simulink subsystem "PvtSubSys_AHBC"  (R2020b)
settings: Solver=VariableStepAuto  StartTime=0.0  StopTime=10.0  RelTol=1e-3
undefined symbols (not defined in the file): P_AHBC_ABS_ENABLE, P_AHBC_DRIVE_DIRECTION_ENABLE, P_AHBC_ESP_ENABLE, P_AHBC_FOG_ENABLE, P_AHBC_FOG_TIME, P_AHBC_HIGHBEAM_ACTIVE_GRACE, P_AHBC_LAT_ACC_ENTER, P_AHBC_LAT_ACC_EXIT, P_AHBC_MAX_ONCOMING_DISTANCE_COUPLE2, P_AHBC_MAX_ONCOMING_DISTANCE_ONE2, P_AHBC_MAX_TAILLIGHT_DISTANCE_COUPLE2, P_AHBC_MAX_TAILLIGHT_DISTANCE_ONE2, P_AHBC_SPEED_SWITCH_HIGH_BEAM_OFF2, P_AHBC_SPEED_SWITCH_HIGH_BEAM_ON2, P_AHBC_TrafficStyle, P_AHBC_TURN_LAMP_ENABLE, P_AHBC_WIPER_ENABLE, P_AHBC_WIPER_TIME, P_AHBC_YAW_RATE_ENTER, P_AHBC_YAW_RATE_EXIT
libraries: simulink x57
(part 1 of 4)
settings Model: Creator=GW00184765  LastModifiedBy=GW00204750

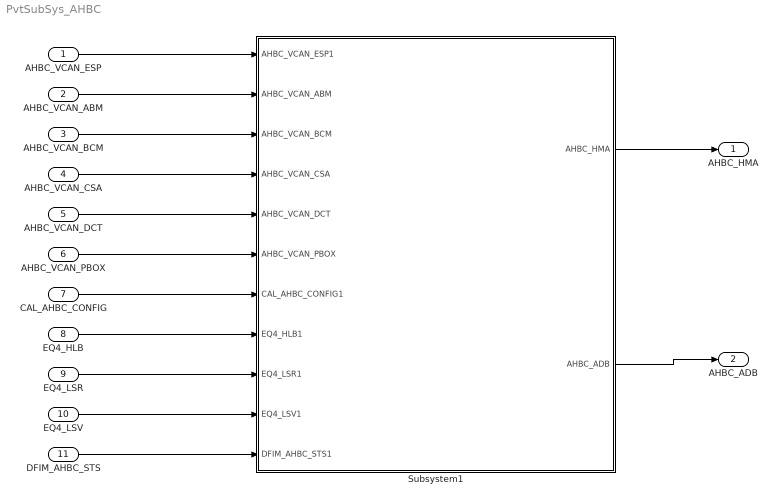
== system PvtSubSys_AHBC ==
  AHBC_VCAN_ESP : Inport  OutDataTypeStr=Bus: VCAN_ESP_MSG_BUS  PortDimensions=1  BusOutputAsStruct=on
  AHBC_VCAN_ABM : Inport  Port=2  OutDataTypeStr=Bus: VCAN_ABM_MSG_BUS  PortDimensions=1  BusOutputAsStruct=on
  AHBC_VCAN_BCM : Inport  Port=3  OutDataTypeStr=Bus: VCAN_BCM_MSG_BUS  PortDimensions=1  BusOutputAsStruct=on
  AHBC_VCAN_CSA : Inport  Port=4  OutDataTypeStr=Bus: VCAN_CSA_MSG_BUS  PortDimensions=1  BusOutputAsStruct=on
  AHBC_VCAN_DCT : Inport  Port=5  OutDataTypeStr=Bus: VCAN_DCT_MSG_BUS  PortDimensions=1  BusOutputAsStruct=on
  AHBC_VCAN_PBOX : Inport  Port=6  OutDataTypeStr=Bus: VCAN_PBOX_MSG_BUS  PortDimensions=1  BusOutputAsStruct=on
  CAL_AHBC_CONFIG : Inport  Port=7  OutDataTypeStr=Bus: CAL_AHBC_CONFIG_BUS  PortDimensions=1  BusOutputAsStruct=on
  EQ4_HLB : Inport  Port=8  OutDataTypeStr=Bus: EQ4_HLB_BUS  PortDimensions=1  BusOutputAsStruct=on
  EQ4_LSR : Inport  Port=9  OutDataTypeStr=Bus: EQ4_LSR_BUS  PortDimensions=1  BusOutputAsStruct=on
  EQ4_LSV : Inport  Port=10  OutDataTypeStr=Bus: EQ4_LSV_BUS  PortDimensions=1  BusOutputAsStruct=on
  DFIM_AHBC_STS : Inport  Port=11  OutDataTypeStr=Bus: DFIM_AHBC_STS_BUS  PortDimensions=1  BusOutputAsStruct=on
  Subsystem1 : Subsystem
  AHBC_HMA : Outport  OutDataTypeStr=Bus: AHBC_HMA_BUS  PortDimensions=1  BusOutputAsStruct=on
  AHBC_ADB : Outport  Port=2  OutDataTypeStr=Bus: AHBC_ADB_BUS  PortDimensions=1  BusOutputAsStruct=on
  wires:
  Subsystem1/2(AHBC_ADB) -> AHBC_ADB/1
  Subsystem1/1(AHBC_HMA) -> AHBC_HMA/1
  AHBC_VCAN_ABM/1 -> Subsystem1/2(AHBC_VCAN_ABM)
  AHBC_VCAN_ESP/1 -> Subsystem1/1(AHBC_VCAN_ESP1)
  AHBC_VCAN_BCM/1 -> Subsystem1/3(AHBC_VCAN_BCM)
  AHBC_VCAN_CSA/1 -> Subsystem1/4(AHBC_VCAN_CSA)
  AHBC_VCAN_DCT/1 -> Subsystem1/5(AHBC_VCAN_DCT)
  AHBC_VCAN_PBOX/1 -> Subsystem1/6(AHBC_VCAN_PBOX)
  CAL_AHBC_CONFIG/1 -> Subsystem1/7(CAL_AHBC_CONFIG1)
  EQ4_HLB/1 -> Subsystem1/8(EQ4_HLB1)
  EQ4_LSR/1 -> Subsystem1/9(EQ4_LSR1)
  EQ4_LSV/1 -> Subsystem1/10(EQ4_LSV1)
  DFIM_AHBC_STS/1 -> Subsystem1/11(DFIM_AHBC_STS1)

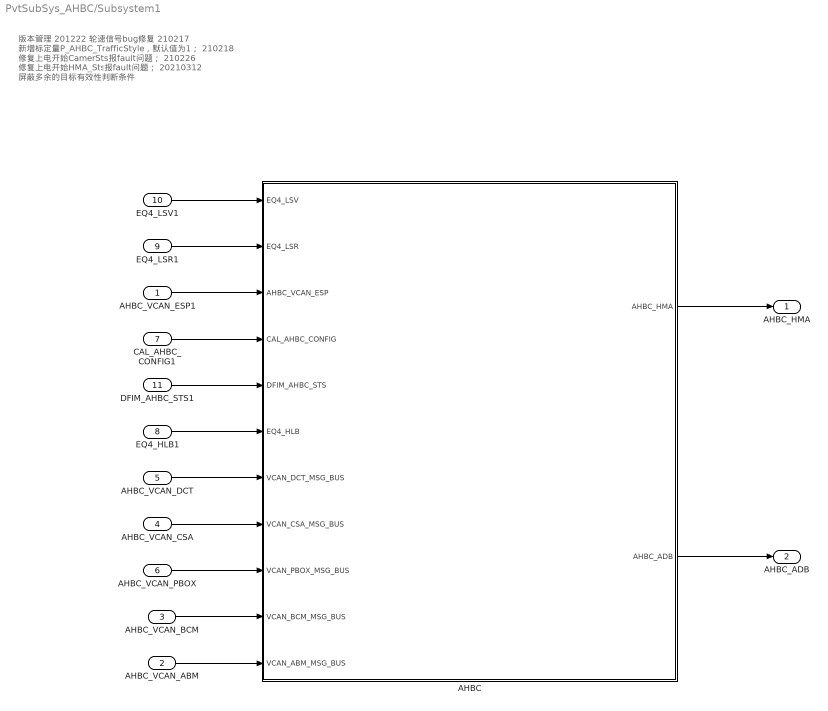
== system PvtSubSys_AHBC/Subsystem1 ==
  note: 版本管理
      | 201222
      | 轮速信号bug修复
      | 210217
      | 新增标定量P_AHBC_TrafficStyle，默认值为1；
      | 210218
      | 修复上电开始CamerSts报fault问题；
      | 210226
      | 修复上电开始HMA_Sts报fault问题；
      | 20210312
      | 屏蔽多余的目标有效性判断条件
  AHBC_VCAN_ESP1 : Inport  OutDataTypeStr=Bus: VCAN_ESP_MSG_BUS  PortDimensions=1  BusOutputAsStruct=on
  AHBC_VCAN_ABM : Inport  Port=2  OutDataTypeStr=Bus: VCAN_ABM_MSG_BUS  PortDimensions=1  BusOutputAsStruct=on
  AHBC_VCAN_BCM : Inport  Port=3  OutDataTypeStr=Bus: VCAN_BCM_MSG_BUS  PortDimensions=1  BusOutputAsStruct=on
  AHBC_VCAN_CSA : Inport  Port=4  OutDataTypeStr=Bus: VCAN_CSA_MSG_BUS  PortDimensions=1  BusOutputAsStruct=on
  AHBC_VCAN_DCT : Inport  Port=5  OutDataTypeStr=Bus: VCAN_DCT_MSG_BUS  PortDimensions=1  BusOutputAsStruct=on
  AHBC_VCAN_PBOX : Inport  Port=6  OutDataTypeStr=Bus: VCAN_PBOX_MSG_BUS  PortDimensions=1  BusOutputAsStruct=on
  CAL_AHBC_CONFIG1 : Inport  Port=7  OutDataTypeStr=Bus: CAL_AHBC_CONFIG_BUS  PortDimensions=1  BusOutputAsStruct=on
  EQ4_HLB1 : Inport  Port=8  OutDataTypeStr=Bus: EQ4_HLB_BUS  PortDimensions=1  BusOutputAsStruct=on
  EQ4_LSR1 : Inport  Port=9  OutDataTypeStr=Bus: EQ4_LSR_BUS  PortDimensions=1  BusOutputAsStruct=on
  EQ4_LSV1 : Inport  Port=10  OutDataTypeStr=Bus: EQ4_LSV_BUS  PortDimensions=1  BusOutputAsStruct=on
  DFIM_AHBC_STS1 : Inport  Port=11  OutDataTypeStr=Bus: DFIM_AHBC_STS_BUS  PortDimensions=1  BusOutputAsStruct=on
  AHBC : Subsystem
  AHBC_HMA : Outport  OutDataTypeStr=Bus: AHBC_HMA_BUS  PortDimensions=1  BusOutputAsStruct=on
  AHBC_ADB : Outport  Port=2  OutDataTypeStr=Bus: AHBC_ADB_BUS  PortDimensions=1  BusOutputAsStruct=on
  wires:
  AHBC/2(AHBC_ADB) -> AHBC_ADB/1
  AHBC/1(AHBC_HMA) -> AHBC_HMA/1
  EQ4_LSV1/1 -> AHBC/1(EQ4_LSV)
  EQ4_LSR1/1 -> AHBC/2(EQ4_LSR)
  EQ4_HLB1/1 -> AHBC/6(EQ4_HLB)
  AHBC_VCAN_ESP1/1 -> AHBC/3(AHBC_VCAN_ESP)
  AHBC_VCAN_ABM/1 -> AHBC/11(VCAN_ABM_MSG_BUS)
  AHBC_VCAN_BCM/1 -> AHBC/10(VCAN_BCM_MSG_BUS)
  AHBC_VCAN_CSA/1 -> AHBC/8(VCAN_CSA_MSG_BUS)
  AHBC_VCAN_DCT/1 -> AHBC/7(VCAN_DCT_MSG_BUS)
  AHBC_VCAN_PBOX/1 -> AHBC/9(VCAN_PBOX_MSG_BUS)
  CAL_AHBC_CONFIG1/1 -> AHBC/4(CAL_AHBC_CONFIG)
  DFIM_AHBC_STS1/1 -> AHBC/5(DFIM_AHBC_STS)

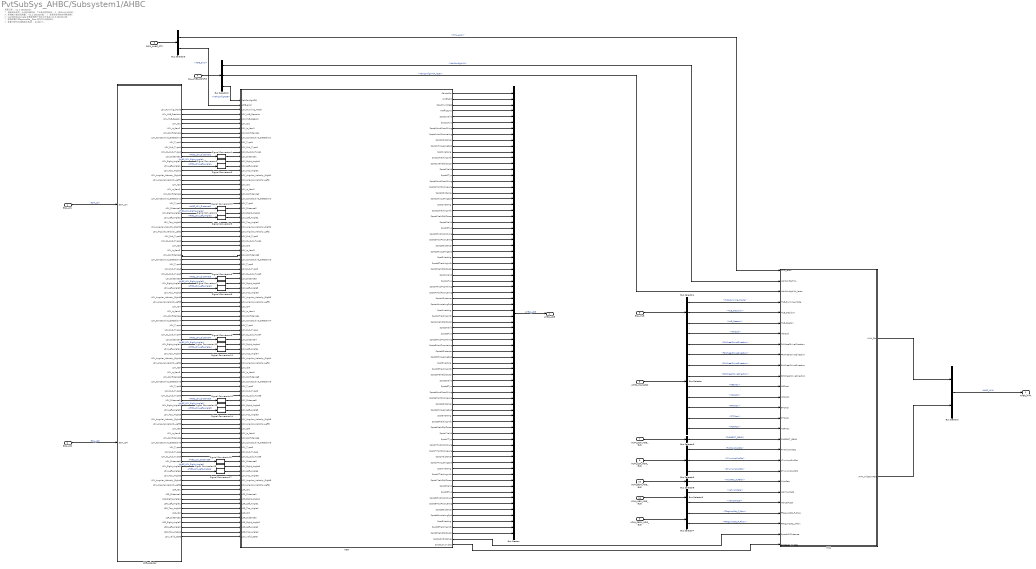
== system PvtSubSys_AHBC/Subsystem1/AHBC ==
  note: 变更记录：
      | V2.1
      | 20201027：
      | 1、调换目标类型，1-6是车辆目标，7-8是反射物目标；
      | 2、修改HMA状态机；
      | 3、新增输入输出观测量；
      | V2.2
      | 20201031：
      | 1、新增目标有效性判断逻辑；
      | 2、LightCtrlParameter字典新增两个自定义的BUS
      | V2.3
      | 20201109：
      | 1、新增后雾灯RFogLmpSts__Pbox信号作为抑制条件；
      | 2、修复行驶方向抑制条件BUG；
      | 210217
      | 新增标定量P_AHBC_TrafficStyle，默认值为1；
      | 210218
      | 修复上电开始CamerSts报fault问题；
      | 210220
      | 优化AmBlight、RoadIllumDetd信号判断逻辑；
      | 210226
      | 修复上电开始HMA_Sts报fault问题；
      | 20210312
      | 屏蔽多余的目标有效性判断条件
  EQ4_LSV : Inport  OutDataTypeStr=Bus: EQ4_LSV_BUS
  EQ4_LSR : Inport  Port=2  OutDataTypeStr=Bus: EQ4_LSR_BUS
  AHBC_VCAN_ESP : Inport  Port=3  OutDataTypeStr=Bus: VCAN_ESP_MSG_BUS  PortDimensions=1  BusOutputAsStruct=on
  CAL_AHBC_CONFIG : Inport  Port=4  OutDataTypeStr=Bus: CAL_AHBC_CONFIG_BUS  PortDimensions=1  BusOutputAsStruct=on
  DFIM_AHBC_STS : Inport  Port=5  OutDataTypeStr=Bus: DFIM_AHBC_STS_BUS  PortDimensions=1  BusOutputAsStruct=on
  EQ4_HLB : Inport  Port=6  OutDataTypeStr=Bus: EQ4_HLB_BUS  PortDimensions=1  BusOutputAsStruct=on
  VCAN_DCT_MSG_BUS : Inport  Port=7  OutDataTypeStr=Bus: VCAN_DCT_MSG_BUS
  VCAN_CSA_MSG_BUS : Inport  Port=8  OutDataTypeStr=Bus: VCAN_CSA_MSG_BUS
  VCAN_PBOX_MSG_BUS : Inport  Port=9  OutDataTypeStr=Bus: VCAN_PBOX_MSG_BUS
  VCAN_BCM_MSG_BUS : Inport  Port=10  OutDataTypeStr=Bus: VCAN_BCM_MSG_BUS
  VCAN_ABM_MSG_BUS : Inport  Port=11  OutDataTypeStr=Bus: VCAN_ABM_MSG_BUS
  ADB : Subsystem
  ADB_adapter : Subsystem
  Bus Creator : BusCreator  Inputs=76  OutDataTypeStr=Bus: AHBC_ADB_BUS
      settings: InheritFromInputs=off
  Bus Creator1 : BusCreator  Inputs=2  OutDataTypeStr=Bus: AHBC_HMA_BUS
  Bus Selector : BusSelector  OutputSignals=VehSpd,FLWheelDriveDirection,FRWheelDriveDirection,RLWheelDriveDirection,RRWheelDriveDirection,ABSActv,VDCActv,BTCActv,PTCActv,MSRActv
  Bus Selector2 : BusSelector  OutputSignals=VehConfigHMA,VehConfigHMA_laser,VehConfigADB
  Bus Selector3 : BusSelector  OutputSignals=HMA_error,ADB_error
  Bus Selector4 : BusSelector  OutputSignals=EQ4_HLB_HDR.HLB_Running_Mode,EQ4_HLB_HDR.HLB_Decision,EQ4_HLB_HDR.HLB_Reason
  Bus Selector5 : BusSelector  OutputSignals=CURRENT_GEAR
  Bus Selector6 : BusSelector  OutputSignals=FrntWiprSwtSts,LTurnLmpSwtSts,RTurnLmpSwtSts
  Bus Selector7 : BusSelector  OutputSignals=FFogLmpSts_F_Pbox,RFogLmpSts_R_Pbox
  Bus Selector8 : BusSelector  OutputSignals=WiprReq_F_PBOX
  Bus Selector9 : BusSelector  OutputSignals=VehYawRate,VehLatAccel
  HMA : Subsystem
  Signal Conversion{1..17,97} (18 alike) : SignalConversion  OverrideOpt=off
  AHBC_HMA : Outport  OutDataTypeStr=Bus: AHBC_HMA_BUS  PortDimensions=1  BusOutputAsStruct=on
  AHBC_ADB : Outport  Port=2  OutDataTypeStr=Bus: AHBC_ADB_BUS  PortDimensions=1  BusOutputAsStruct=on
  wires:
  ADB_adapter/92(LSV_valid_state) -> ADB/94(LSV_valid_state)
  Bus Selector9/2 -> HMA/23(VehLatAccel)  "<VehLatAccel>"
  Bus Selector9/1 -> HMA/22(VehYawRate)  "<VehYawRate>"
  VCAN_ABM_MSG_BUS/1 -> Bus Selector9/1
  Bus Selector8/1 -> HMA/21(WiprReq)  "<WiprReq_F_PBOX>"
  VCAN_BCM_MSG_BUS/1 -> Bus Selector8/1
  Bus Selector7/2 -> HMA/25(RFogLmpSts__Pbox)  "<RFogLmpSts_R_Pbox>"
  Bus Selector7/1 -> HMA/24(FFogLmpSts_F_Pbox)  "<FFogLmpSts_F_Pbox>"
  VCAN_PBOX_MSG_BUS/1 -> Bus Selector7/1
  Bus Selector6/3 -> HMA/20(RTurnLmpSwtSts)  "<RTurnLmpSwtSts>"
  Bus Selector6/2 -> HMA/19(LTurnLmpSwtSts)  "<LTurnLmpSwtSts>"
  Bus Selector6/1 -> HMA/18(FrntWiprSwtSts)  "<FrntWiprSwtSts>"
  VCAN_CSA_MSG_BUS/1 -> Bus Selector6/1
  Bus Selector5/1 -> HMA/17(CURRENT_GEAR)  "<CURRENT_GEAR>"
  VCAN_DCT_MSG_BUS/1 -> Bus Selector5/1
  Signal Conversion17/1 -> ADB/80(LSV_Left_Angle6)
  Signal Conversion16/1 -> ADB/79(LSV_Right_Angle6)
  Signal Conversion15/1 -> ADB/78(LSV_Distance6)
  Signal Conversion14/1 -> ADB/67(LSV_Left_Angle5)
  Signal Conversion13/1 -> ADB/66(LSV_Right_Angle5)
  Signal Conversion12/1 -> ADB/65(LSV_Distance5)
  Signal Conversion11/1 -> ADB/54(LSV_Left_Angle4)
  Signal Conversion10/1 -> ADB/53(LSV_Right_Angle4)
  Signal Conversion9/1 -> ADB/52(LSV_Distance4)
  Signal Conversion8/1 -> ADB/41(LSV_Left_Angle3)
  Signal Conversion7/1 -> ADB/40(LSV_Right_Angle3)
  Signal Conversion6/1 -> ADB/39(LSV_Distance3)
  Signal Conversion5/1 -> ADB/26(LSV_Left_Angle2)
  Signal Conversion4/1 -> ADB/25(LSV_Right_Angle2)
  Signal Conversion3/1 -> ADB/15(LSV_Left_Angle1)
  Signal Conversion2/1 -> ADB/14(LSV_Right_Angle1)
  Signal Conversion1/1 -> ADB/13(LSV_Distance1)
  Signal Conversion97/1 -> ADB/24(LSV_Distance2)
  ADB_adapter/91(LSR_Top_Angle2) -> ADB/93(LSR_Top_Angle2)
  ADB_adapter/90(LSR_Left_Angle2) -> ADB/92(LSR_Left_Angle2)
  ADB_adapter/89(LSR_Right_Angle2) -> ADB/91(LSR_Right_Angle2)
  ADB_adapter/88(LSR_Distance2) -> ADB/90(LSR_Distance2)
  ADB_adapter/87(LSR_ID2) -> ADB/89(LSR_ID2)
  ADB_adapter/86(LSR_Top_Angle1) -> ADB/88(LSR_Top_Angle1)
  ADB_adapter/85(LSR_Left_Angle1) -> ADB/87(LSR_Left_Angle1)
  ADB_adapter/84(LSR_Right_Angle1) -> ADB/86(LSR_Right_Angle1)
  ADB_adapter/83(LSR_Distance1) -> ADB/85(LSR_Distance1)
  ADB_adapter/82(LSR_ID1) -> ADB/84(LSR_ID1)
  ADB_adapter/81(LSV_Angular_Velocity_Left6) -> ADB/83(LSV_Angular_Velocity_Left6)
  ADB_adapter/80(LSV_Angular_Velocity_Right6) -> ADB/82(LSV_Angular_Velocity_Right6)
  ADB_adapter/79(LSV_Top_Angle6) -> ADB/81(LSV_Top_Angle6)
  ADB_adapter/78(LSV_Left_Angle6) -> Signal Conversion17/1  "AHBC_LSV_Left_Angle6"
  ADB_adapter/77(LSV_Right_Angle6) -> Signal Conversion16/1  "AHBC_LSV_Right_Angle6"
  ADB_adapter/76(LSV_Distance6) -> Signal Conversion15/1  "AHBC_LSV_Distance6"
  ADB_adapter/75(LSV_CL_Sub_Type6) -> ADB/77(LSV_CL_Sub_Type6)
  ADB_adapter/74(LSV_Sub_Type6) -> ADB/76(LSV_Sub_Type6)
  ADB_adapter/73(LSV_Type6) -> ADB/75(LSV_Type6)
  ADB_adapter/72(LSV_Consecutive_Detection6) -> ADB/74(LSV_Consecutive_Detection6)
  ADB_adapter/71(LSV_Confidence6) -> ADB/73(LSV_Confidence6)
  ADB_adapter/70(LSV_Is_New6) -> ADB/72(LSV_Is_New6)
  ADB_adapter/69(LSV_ID6) -> ADB/71(LSV_ID6)
  ADB_adapter/68(LSV_Angular_Velocity_Left5) -> ADB/70(LSV_Angular_Velocity_Left5)
  ADB_adapter/67(LSV_Angular_Velocity_Right5) -> ADB/69(LSV_Angular_Velocity_Right5)
  ADB_adapter/66(LSV_Top_Angle5) -> ADB/68(LSV_Top_Angle5)
  ADB_adapter/65(LSV_Left_Angle5) -> Signal Conversion14/1  "AHBC_LSV_Left_Angle5"
  ADB_adapter/64(LSV_Right_Angle5) -> Signal Conversion13/1  "AHBC_LSV_Right_Angle5"
  ADB_adapter/63(LSV_Distance5) -> Signal Conversion12/1  "AHBC_LSV_Distance5"
  ADB_adapter/62(LSV_CL_Sub_Type5) -> ADB/64(LSV_CL_Sub_Type5)
  ADB_adapter/61(LSV_Sub_Type5) -> ADB/63(LSV_Sub_Type5)
  ADB_adapter/60(LSV_Type5) -> ADB/62(LSV_Type5)
  ADB_adapter/59(LSV_Consecutive_Detection5) -> ADB/61(LSV_Consecutive_Detection5)
  ADB_adapter/58(LSV_Confidence5) -> ADB/60(LSV_Confidence5)
  ADB_adapter/57(LSV_Is_New5) -> ADB/59(LSV_Is_New5)
  ADB_adapter/56(LSV_ID5) -> ADB/58(LSV_ID5)
  ADB_adapter/55(LSV_Angular_Velocity_Left4) -> ADB/57(LSV_Angular_Velocity_Left4)
  ADB_adapter/54(LSV_Angular_Velocity_Right4) -> ADB/56(LSV_Angular_Velocity_Right4)
  ADB_adapter/53(LSV_Top_Angle4) -> ADB/55(LSV_Top_Angle4)
  ADB_adapter/52(LSV_Left_Angle4) -> Signal Conversion11/1  "AHBC_LSV_Left_Angle4"
  ADB_adapter/51(LSV_Right_Angle4) -> Signal Conversion10/1  "AHBC_LSV_Right_Angle4"
  ADB_adapter/50(LSV_Distance4) -> Signal Conversion9/1  "AHBC_LSV_Distance4"
  ADB_adapter/49(LSV_CL_Sub_Type4) -> ADB/51(LSV_CL_Sub_Type4)
  ADB_adapter/48(LSV_Sub_Type4) -> ADB/50(LSV_Sub_Type4)
  ADB_adapter/47(LSV_Type4) -> ADB/49(LSV_Type4)
  ADB_adapter/46(LSV_Consecutive_Detection4) -> ADB/48(LSV_Consecutive_Detection4)
  ADB_adapter/45(LSV_Confidence4) -> ADB/47(LSV_Confidence4)
  ADB_adapter/44(LSV_Is_New4) -> ADB/46(LSV_Is_New4)
  ADB_adapter/43(LSV_ID4) -> ADB/45(LSV_ID4)
  ADB_adapter/42(LSV_Angular_Velocity_Left3) -> ADB/44(LSV_Angular_Velocity_Left3)
  ADB_adapter/41(LSV_Angular_Velocity_Right3) -> ADB/43(LSV_Angular_Velocity_Right3)
  ADB_adapter/40(LSV_Top_Angle3) -> ADB/42(LSV_Top_Angle3)
  ADB_adapter/39(LSV_Left_Angle3) -> Signal Conversion8/1  "AHBC_LSV_Left_Angle3"
  ADB_adapter/38(LSV_Right_Angle3) -> Signal Conversion7/1  "AHBC_LSV_Right_Angle3"
  ADB_adapter/37(LSV_Distance3) -> Signal Conversion6/1  "AHBC_LSV_Distance3"
  ADB_adapter/36(LSV_CL_Sub_Type3) -> ADB/38(LSV_CL_Sub_Type3)
  ADB_adapter/35(LSV_Sub_Type3) -> ADB/37(LSV_Sub_Type3)
  ADB_adapter/34(LSV_Type3) -> ADB/36(LSV_Type3)
  ADB_adapter/33(LSV_Consecutive_Detection3) -> ADB/35(LSV_Consecutive_Detection3)
  ADB_adapter/32(LSV_Confidence3) -> ADB/34(LSV_Confidence3)
  ADB_adapter/31(LSV_Is_New3) -> ADB/33(LSV_Is_New3)
  ADB_adapter/30(LSV_ID3) -> ADB/32(LSV_ID3)
  ADB_adapter/29(LSV_CL_Sub_Type2) -> ADB/31(LSV_CL_Sub_Type2)
  ADB_adapter/28(LSV_Sub_Type2) -> ADB/30(LSV_Sub_Type2)
  ADB_adapter/27(LSV_Angular_Velocity_Left2) -> ADB/29(LSV_Angular_Velocity_Left2)
  ADB_adapter/26(LSV_Angular_Velocity_Right2) -> ADB/28(LSV_Angular_Velocity_Right2)
  ADB_adapter/25(LSV_Top_Angle2) -> ADB/27(LSV_Top_Angle2)
  ADB_adapter/24(LSV_Left_Angle2) -> Signal Conversion5/1  "AHBC_LSV_Left_Angle2"
  ADB_adapter/23(LSV_Right_Angle2) -> Signal Conversion4/1  "AHBC_LSV_Right_Angle2"
  ADB_adapter/22(LSV_Distance2) -> Signal Conversion97/1  "AHBC_LSV_Distance2"
  ADB_adapter/21(LSV_Type2) -> ADB/23(LSV_Type2)
  ADB_adapter/20(LSV_Consecutive_Detection2) -> ADB/22(LSV_Consecutive_Detection2)
  ADB_adapter/19(LSV_Confidence2) -> ADB/21(LSV_Confidence2)
  ADB_adapter/18(LSV_Is_New2) -> ADB/20(LSV_Is_New2)
  ADB_adapter/17(LSV_ID2) -> ADB/19(LSV_ID2)
  ADB_adapter/16(LSV_Angular_Velocity_Left1) -> ADB/18(LSV_Angular_Velocity_Left1)
  ADB_adapter/15(LSV_Angular_Velocity_Right1) -> ADB/17(LSV_Angular_Velocity_Right1)
  ADB_adapter/14(LSV_Top_Angle1) -> ADB/16(LSV_Top_Angle1)
  ADB_adapter/13(LSV_Left_Angle1) -> Signal Conversion3/1  "AHBC_LSV_Left_Angle1"
  ADB_adapter/12(LSV_Right_Angle1) -> Signal Conversion2/1  "AHBC_LSV_Right_Angle1"
  ADB_adapter/11(LSV_Distance1) -> Signal Conversion1/1  "AHBC_LSV_Distance1"
  ADB_adapter/10(LSV_CL_Sub_Type1) -> ADB/12(LSV_CL_Sub_Type1)
  ADB_adapter/9(LSV_Sub_Type1) -> ADB/11(LSV_Sub_Type1)
  ADB_adapter/8(LSV_Type1) -> ADB/10(LSV_Type1)
  ADB_adapter/7(LSV_Consecutive_Detection1) -> ADB/9(LSV_Consecutive_Detection1)
  ADB_adapter/6(LSV_Confidence1) -> ADB/8(LSV_Confidence1)
  ADB_adapter/5(LSV_Is_New1) -> ADB/7(LSV_Is_New1)
  ADB_adapter/4(LSV_ID1) -> ADB/6(LSV_ID1)
  ADB_adapter/3(LSV_HLB_Reason) -> ADB/5(LSV_HLB_Reason)
  ADB_adapter/2(LSV_HLB_Decision) -> ADB/4(LSV_HLB_Decision)
  ADB_adapter/1(LSV_Running_Mode) -> ADB/3(LSV_Running_Mode)
  ADB/76(Spots8VehObjClassn) -> Bus Creator/76
  ADB/75(Spots8TrackingInfo) -> Bus Creator/75
  ADB/74(Spot8VertAng) -> Bus Creator/74
  ADB/73(Spots8HozLeAngSpd) -> Bus Creator/73
  ADB/72(Spots8Distance) -> Bus Creator/72
  ADB/71(Spots8HozlPosnLeAng) -> Bus Creator/71
  ADB/70(Spots8HozlPosnRiAng) -> Bus Creator/70
  ADB/69(Spots8Typ) -> Bus Creator/69
  ADB/68(Spots8Valid) -> Bus Creator/68
  ADB/67(Spots7VehObjClassn) -> Bus Creator/67
  ADB/66(Spots7TrackingInfo) -> Bus Creator/66
  ADB/65(Spot7VertAng) -> Bus Creator/65
  ADB/64(Spots7HozLeAngSpd) -> Bus Creator/64
  ADB/63(Spots7Distance) -> Bus Creator/63
  ADB/62(Spots7HozlPosnLeAng) -> Bus Creator/62
  ADB/61(Spots7HozlPosnRiAng) -> Bus Creator/61
  ADB/60(Spots7Typ) -> Bus Creator/60
  ADB/59(Spots7Valid) -> Bus Creator/59
  ADB/58(Spots6VehObjClassn) -> Bus Creator/58
  ADB/57(Spots6TrackingInfo) -> Bus Creator/57
  ADB/56(Spot6VertAng) -> Bus Creator/56
  ADB/55(Spots6HozLeAngSpd) -> Bus Creator/55
  ADB/54(Spots6Distance) -> Bus Creator/54
  ADB/53(Spots6HozlPosnLeAng) -> Bus Creator/53
  ADB/52(Spots6HozlPosnRiAng) -> Bus Creator/52
  ADB/51(Spots6Typ) -> Bus Creator/51
  ADB/50(Spots6Valid) -> Bus Creator/50
  ADB/49(Spots5VehObjClassn) -> Bus Creator/49
  ADB/48(Spots5TrackingInfo) -> Bus Creator/48
  ADB/47(Spot5VertAng) -> Bus Creator/47
  ADB/46(Spots5HozLeAngSpd) -> Bus Creator/46
  ADB/45(Spots5Distance) -> Bus Creator/45
  ADB/44(Spots5HozlPosnLeAng) -> Bus Creator/44
  ADB/43(Spots5HozlPosnRiAng) -> Bus Creator/43
  ADB/42(Spots5Typ) -> Bus Creator/42
  ADB/41(Spots5Valid) -> Bus Creator/41
  ADB/40(Spots4VehObjClassn) -> Bus Creator/40
  ADB/39(Spots4TrackingInfo) -> Bus Creator/39
  ADB/38(Spot4VertAng) -> Bus Creator/38
  ADB/37(Spots4HozLeAngSpd) -> Bus Creator/37
  ADB/36(Spots4Distance) -> Bus Creator/36
  ADB/35(Spots4HozlPosnLeAng) -> Bus Creator/35
  ADB/34(Spots4HozlPosnRiAng) -> Bus Creator/34
  ADB/33(Spots4Typ) -> Bus Creator/33
  ADB/32(Spots4Valid) -> Bus Creator/32
  ADB/31(Spots3VehObjClassn) -> Bus Creator/31
  ADB/30(Spots3TrackingInfo) -> Bus Creator/30
  ADB/29(Spot3VertAng) -> Bus Creator/29
  ADB/28(Spots3HozLeAngSpd) -> Bus Creator/28
  ADB/27(Spots3Distance) -> Bus Creator/27
  ADB/26(Spots3HozlPosnLeAng) -> Bus Creator/26
  ADB/25(Spots3HozlPosnRiAng) -> Bus Creator/25
  ADB/24(Spots3Typ) -> Bus Creator/24
  ADB/23(Spots3Valid) -> Bus Creator/23
  ADB/22(Spots2VehObjClassn) -> Bus Creator/22
  ADB/21(Spots2TrackingInfo) -> Bus Creator/21
  ADB/20(Spot2VertAng) -> Bus Creator/20
  ADB/19(Spots2HozLeAngSpd) -> Bus Creator/19
  ADB/18(Spots2Distance) -> Bus Creator/18
  ADB/17(Spots2HozlPosnLeAng) -> Bus Creator/17
  ADB/16(Spots2HozlPosnRiAng) -> Bus Creator/16
  ADB/15(Spots2Typ) -> Bus Creator/15
  ADB/14(Spots2Valid) -> Bus Creator/14
  ADB/13(Spots1VehObjClassn) -> Bus Creator/13
  ADB/12(Spots1TrackingInfo) -> Bus Creator/12
  ADB/11(Spot1VertAng) -> Bus Creator/11
  ADB/10(Spots1HozLeAngSpd) -> Bus Creator/10
  ADB/9(Spots1Distance) -> Bus Creator/9
  ADB/8(Spots1HozlPosnLeAng) -> Bus Creator/8
  ADB/7(Spots1HozlPosnRiAng) -> Bus Creator/7
  ADB/6(Spots1Typ) -> Bus Creator/6
  ADB/5(Spots1Valid) -> Bus Creator/5
  ADB/4(Trafficstyle) -> Bus Creator/4
  ADB/3(RoadIllumDetd) -> Bus Creator/3
  ADB/2(AmBlight) -> Bus Creator/2
  ADB/1(CamerSts) -> Bus Creator/1
  Bus Selector4/2 -> HMA/5(HLB_Decision)  "<HLB_Decision>"
  Bus Selector4/1 -> HMA/4(HLB_Running_Mode)  "<HLB_Running_Mode>"
  EQ4_HLB/1 -> Bus Selector4/1
  Bus Selector4/3 -> HMA/6(HLB_Reason)  "<HLB_Reason>"
  Bus Selector3/1 -> HMA/1(HMA_error)  "<HMA_error>"
  DFIM_AHBC_STS/1 -> Bus Selector3/1
  Bus Selector2/1 -> HMA/2(VehConfigHMA)  "<VehConfigHMA>"
  Bus Selector2/2 -> HMA/3(VehConfigHMA_laser)  "<VehConfigHMA_laser>"
  CAL_AHBC_CONFIG/1 -> Bus Selector2/1
  Bus Selector/9 -> HMA/15(PTCActv)  "<PTCActv>"
  Bus Selector/8 -> HMA/14(BTCActv)  "<BTCActv>"
  Bus Selector/7 -> HMA/13(VDCActv)  "<VDCActv>"
  Bus Selector/6 -> HMA/12(ABSActv)  "<ABSActv>"
  Bus Selector/10 -> HMA/16(MSRActv)  "<MSRActv>"
  AHBC_VCAN_ESP/1 -> Bus Selector/1
  ADB/78(SpotsLSV_Types) -> HMA/27(SpotsLSV_Types)
  ADB/77(SpotsLSVDistance) -> HMA/26(SpotsLSVDistance)
  Bus Creator1/1 -> AHBC_HMA/1  "AHBC_HMA"
  Bus Creator/1 -> AHBC_ADB/1  "AHBC_ADB"
  Bus Selector/1 -> HMA/7(VehSpd)  "<VehSpd>"
  Bus Selector/5 -> HMA/11(RRWheelDriveDirection)  "<RRWheelDriveDirection>"
  Bus Selector/4 -> HMA/10(RLWheelDriveDirection)  "<RLWheelDriveDirection>"
  Bus Selector/3 -> HMA/9(FRWheelDriveDirection)  "<FRWheelDriveDirection>"
  Bus Selector/2 -> HMA/8(FLWheelDriveDirection)  "<FLWheelDriveDirection>"
  Bus Selector3/2 -> ADB/2(ADB_error)  "<ADB_error>"
  EQ4_LSV/1 -> ADB_adapter/1(EQ4_LSV)  "EQ4_LSV"
  EQ4_LSR/1 -> ADB_adapter/2(EQ4_LSR)  "EQ4_LSR"
  Bus Selector2/3 -> ADB/1(VehConfigADB)  "<VehConfigADB>"
  HMA/2(HMA_HibeamReq) -> Bus Creator1/2
  HMA/1(HMA_Sts) -> Bus Creator1/1

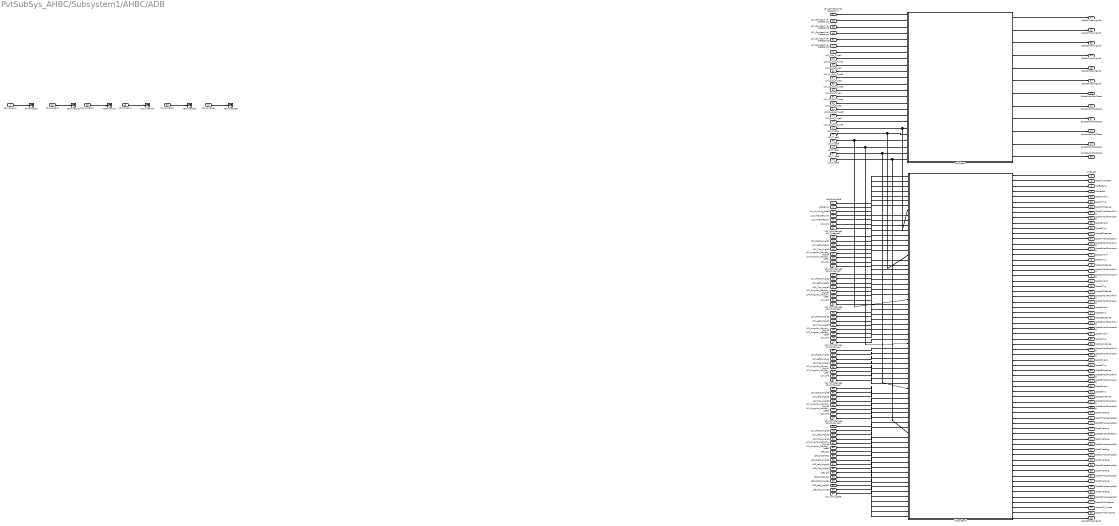
== system PvtSubSys_AHBC/Subsystem1/AHBC/ADB ==
  VehConfigADB : Inport
  ADB_error : Inport  Port=2
  LSV_Running_Mode : Inport  Port=3
  LSV_HLB_Decision : Inport  Port=4
  LSV_HLB_Reason : Inport  Port=5
  LSV_ID1 : Inport  Port=6
  LSV_Is_New1 : Inport  Port=7
  LSV_Confidence1 : Inport  Port=8
  LSV_Consecutive_Detection1 : Inport  Port=9
  LSV_Type1 : Inport  Port=10
  LSV_Sub_Type1 : Inport  Port=11
  LSV_CL_Sub_Type1 : Inport  Port=12
  LSV_Distance1 : Inport  Port=13  OutDataTypeStr=uint16
  LSV_Right_Angle1 : Inport  Port=14
  LSV_Left_Angle1 : Inport  Port=15
  LSV_Top_Angle1 : Inport  Port=16
  LSV_Angular_Velocity_Right1 : Inport  Port=17
  LSV_Angular_Velocity_Left1 : Inport  Port=18
  LSV_ID2 : Inport  Port=19
  LSV_Is_New2 : Inport  Port=20
  LSV_Confidence2 : Inport  Port=21
  LSV_Consecutive_Detection2 : Inport  Port=22
  LSV_Type2 : Inport  Port=23
  LSV_Distance2 : Inport  Port=24  OutDataTypeStr=uint16
  LSV_Right_Angle2 : Inport  Port=25
  LSV_Left_Angle2 : Inport  Port=26
  LSV_Top_Angle2 : Inport  Port=27
  LSV_Angular_Velocity_Right2 : Inport  Port=28
  LSV_Angular_Velocity_Left2 : Inport  Port=29
  LSV_Sub_Type2 : Inport  Port=30
  LSV_CL_Sub_Type2 : Inport  Port=31
  LSV_ID3 : Inport  Port=32
  LSV_Is_New3 : Inport  Port=33
  LSV_Confidence3 : Inport  Port=34
  LSV_Consecutive_Detection3 : Inport  Port=35
  LSV_Type3 : Inport  Port=36
  LSV_Sub_Type3 : Inport  Port=37
  LSV_CL_Sub_Type3 : Inport  Port=38
  LSV_Distance3 : Inport  Port=39  OutDataTypeStr=uint16
  LSV_Right_Angle3 : Inport  Port=40
  LSV_Left_Angle3 : Inport  Port=41
  LSV_Top_Angle3 : Inport  Port=42
  LSV_Angular_Velocity_Right3 : Inport  Port=43
  LSV_Angular_Velocity_Left3 : Inport  Port=44
  LSV_ID4 : Inport  Port=45
  LSV_Is_New4 : Inport  Port=46
  LSV_Confidence4 : Inport  Port=47
  LSV_Consecutive_Detection4 : Inport  Port=48
  LSV_Type4 : Inport  Port=49
  LSV_Sub_Type4 : Inport  Port=50
  LSV_CL_Sub_Type4 : Inport  Port=51
  LSV_Distance4 : Inport  Port=52  OutDataTypeStr=uint16
  LSV_Right_Angle4 : Inport  Port=53
  LSV_Left_Angle4 : Inport  Port=54
  LSV_Top_Angle4 : Inport  Port=55
  LSV_Angular_Velocity_Right4 : Inport  Port=56
  LSV_Angular_Velocity_Left4 : Inport  Port=57
  LSV_ID5 : Inport  Port=58
  LSV_Is_New5 : Inport  Port=59
  LSV_Confidence5 : Inport  Port=60
  LSV_Consecutive_Detection5 : Inport  Port=61
  LSV_Type5 : Inport  Port=62
  LSV_Sub_Type5 : Inport  Port=63
  LSV_CL_Sub_Type5 : Inport  Port=64
  LSV_Distance5 : Inport  Port=65  OutDataTypeStr=uint16
  LSV_Right_Angle5 : Inport  Port=66
  LSV_Left_Angle5 : Inport  Port=67
  LSV_Top_Angle5 : Inport  Port=68
  LSV_Angular_Velocity_Right5 : Inport  Port=69
  LSV_Angular_Velocity_Left5 : Inport  Port=70
  LSV_ID6 : Inport  Port=71
  LSV_Is_New6 : Inport  Port=72
  LSV_Confidence6 : Inport  Port=73
  LSV_Consecutive_Detection6 : Inport  Port=74
  LSV_Type6 : Inport  Port=75
  LSV_Sub_Type6 : Inport  Port=76
  LSV_CL_Sub_Type6 : Inport  Port=77
  LSV_Distance6 : Inport  Port=78  OutDataTypeStr=uint16
  LSV_Right_Angle6 : Inport  Port=79
  LSV_Left_Angle6 : Inport  Port=80
  LSV_Top_Angle6 : Inport  Port=81
  LSV_Angular_Velocity_Right6 : Inport  Port=82
  LSV_Angular_Velocity_Left6 : Inport  Port=83
  LSR_ID1 : Inport  Port=84
  LSR_Distance1 : Inport  Port=85  OutDataTypeStr=uint16
  LSR_Right_Angle1 : Inport  Port=86
  LSR_Left_Angle1 : Inport  Port=87
  LSR_Top_Angle1 : Inport  Port=88
  LSR_ID2 : Inport  Port=89
  LSR_Distance2 : Inport  Port=90  OutDataTypeStr=uint16
  LSR_Right_Angle2 : Inport  Port=91
  LSR_Left_Angle2 : Inport  Port=92
  LSR_Top_Angle2 : Inport  Port=93
  LSV_valid_state : Inport  Port=94
  ObjClassn : Subsystem
  Subsystem1 : Subsystem
  Terminator{3,10,17,24,31,38} (6 alike) : Terminator
  CamerSts : Outport  OutDataTypeStr=uint8  PortDimensions=1
  AmBlight : Outport  Port=2  OutDataTypeStr=boolean  PortDimensions=1
  RoadIllumDetd : Outport  Port=3  OutDataTypeStr=boolean  PortDimensions=1
  Trafficstyle : Outport  Port=4  OutDataTypeStr=uint8  PortDimensions=1
  Spots1Valid : Outport  Port=5  OutDataTypeStr=boolean  PortDimensions=1
  Spots1Typ : Outport  Port=6  OutDataTypeStr=uint8  PortDimensions=1
  Spots1HozlPosnRiAng : Outport  Port=7  OutDataTypeStr=single  PortDimensions=1
  Spots1HozlPosnLeAng : Outport  Port=8  OutDataTypeStr=single  PortDimensions=1
  Spots1Distance : Outport  Port=9  OutDataTypeStr=uint16  PortDimensions=1
  Spots1HozLeAngSpd : Outport  Port=10  OutDataTypeStr=single  PortDimensions=1
  Spot1VertAng : Outport  Port=11  OutDataTypeStr=single  PortDimensions=1
  Spots1TrackingInfo : Outport  Port=12  OutDataTypeStr=boolean  PortDimensions=1
  Spots1VehObjClassn : Outport  Port=13  OutDataTypeStr=uint8  PortDimensions=1
  Spots2Valid : Outport  Port=14  OutDataTypeStr=boolean  PortDimensions=1
  Spots2Typ : Outport  Port=15  OutDataTypeStr=uint8  PortDimensions=1
  Spots2HozlPosnRiAng : Outport  Port=16  OutDataTypeStr=single  PortDimensions=1
  Spots2HozlPosnLeAng : Outport  Port=17  OutDataTypeStr=single  PortDimensions=1
  Spots2Distance : Outport  Port=18  OutDataTypeStr=uint16  PortDimensions=1
  Spots2HozLeAngSpd : Outport  Port=19  OutDataTypeStr=single  PortDimensions=1
  Spot2VertAng : Outport  Port=20  OutDataTypeStr=single  PortDimensions=1
  Spots2TrackingInfo : Outport  Port=21  OutDataTypeStr=boolean  PortDimensions=1
  Spots2VehObjClassn : Outport  Port=22  OutDataTypeStr=uint8  PortDimensions=1
  Spots3Valid : Outport  Port=23  OutDataTypeStr=boolean  PortDimensions=1
  Spots3Typ : Outport  Port=24  OutDataTypeStr=uint8  PortDimensions=1
  Spots3HozlPosnRiAng : Outport  Port=25  OutDataTypeStr=single  PortDimensions=1
  Spots3HozlPosnLeAng : Outport  Port=26  OutDataTypeStr=single  PortDimensions=1
  Spots3Distance : Outport  Port=27  OutDataTypeStr=uint16  PortDimensions=1
  Spots3HozLeAngSpd : Outport  Port=28  OutDataTypeStr=single  PortDimensions=1
  Spot3VertAng : Outport  Port=29  OutDataTypeStr=single  PortDimensions=1
  Spots3TrackingInfo : Outport  Port=30  OutDataTypeStr=boolean  PortDimensions=1
  Spots3VehObjClassn : Outport  Port=31  OutDataTypeStr=uint8  PortDimensions=1
  Spots4Valid : Outport  Port=32  OutDataTypeStr=boolean  PortDimensions=1
  Spots4Typ : Outport  Port=33  OutDataTypeStr=uint8  PortDimensions=1
  Spots4HozlPosnRiAng : Outport  Port=34  OutDataTypeStr=single  PortDimensions=1
  Spots4HozlPosnLeAng : Outport  Port=35  OutDataTypeStr=single  PortDimensions=1
  Spots4Distance : Outport  Port=36  OutDataTypeStr=uint16  PortDimensions=1
  Spots4HozLeAngSpd : Outport  Port=37  OutDataTypeStr=single  PortDimensions=1
  Spot4VertAng : Outport  Port=38  OutDataTypeStr=single  PortDimensions=1
  Spots4TrackingInfo : Outport  Port=39  OutDataTypeStr=boolean  PortDimensions=1
  Spots4VehObjClassn : Outport  Port=40  OutDataTypeStr=uint8  PortDimensions=1
  Spots5Valid : Outport  Port=41  OutDataTypeStr=boolean  PortDimensions=1
  Spots5Typ : Outport  Port=42  OutDataTypeStr=uint8  PortDimensions=1
  Spots5HozlPosnRiAng : Outport  Port=43  OutDataTypeStr=single  PortDimensions=1
  Spots5HozlPosnLeAng : Outport  Port=44  OutDataTypeStr=single  PortDimensions=1
  Spots5Distance : Outport  Port=45  OutDataTypeStr=uint16  PortDimensions=1
  Spots5HozLeAngSpd : Outport  Port=46  OutDataTypeStr=single  PortDimensions=1
  Spot5VertAng : Outport  Port=47  OutDataTypeStr=single  PortDimensions=1
  Spots5TrackingInfo : Outport  Port=48  OutDataTypeStr=boolean  PortDimensions=1
  Spots5VehObjClassn : Outport  Port=49  OutDataTypeStr=uint8  PortDimensions=1
  Spots6Valid : Outport  Port=50  OutDataTypeStr=boolean  PortDimensions=1
  Spots6Typ : Outport  Port=51  OutDataTypeStr=uint8  PortDimensions=1
  Spots6HozlPosnRiAng : Outport  Port=52  OutDataTypeStr=single  PortDimensions=1
  Spots6HozlPosnLeAng : Outport  Port=53  OutDataTypeStr=single  PortDimensions=1
  Spots6Distance : Outport  Port=54  OutDataTypeStr=uint16  PortDimensions=1
  Spots6HozLeAngSpd : Outport  Port=55  OutDataTypeStr=single  PortDimensions=1
  Spot6VertAng : Outport  Port=56  OutDataTypeStr=single  PortDimensions=1
  Spots6TrackingInfo : Outport  Port=57  OutDataTypeStr=boolean  PortDimensions=1
  Spots6VehObjClassn : Outport  Port=58  OutDataTypeStr=uint8  PortDimensions=1
  Spots7Valid : Outport  Port=59  OutDataTypeStr=boolean  PortDimensions=1
  Spots7Typ : Outport  Port=60  OutDataTypeStr=uint8  PortDimensions=1
  Spots7HozlPosnRiAng : Outport  Port=61  OutDataTypeStr=single  PortDimensions=1
  Spots7HozlPosnLeAng : Outport  Port=62  OutDataTypeStr=single  PortDimensions=1
  Spots7Distance : Outport  Port=63  OutDataTypeStr=uint16  PortDimensions=1
  Spots7HozLeAngSpd : Outport  Port=64  OutDataTypeStr=single  PortDimensions=1
  Spot7VertAng : Outport  Port=65  OutDataTypeStr=single  PortDimensions=1
  Spots7TrackingInfo : Outport  Port=66  OutDataTypeStr=boolean  PortDimensions=1
  Spots7VehObjClassn : Outport  Port=67  OutDataTypeStr=uint8  PortDimensions=1
  Spots8Valid : Outport  Port=68  OutDataTypeStr=boolean  PortDimensions=1
  Spots8Typ : Outport  Port=69  OutDataTypeStr=uint8  PortDimensions=1
  Spots8HozlPosnRiAng : Outport  Port=70  OutDataTypeStr=single  PortDimensions=1
  Spots8HozlPosnLeAng : Outport  Port=71  OutDataTypeStr=single  PortDimensions=1
  Spots8Distance : Outport  Port=72  OutDataTypeStr=uint16  PortDimensions=1
  Spots8HozLeAngSpd : Outport  Port=73  OutDataTypeStr=single  PortDimensions=1
  Spot8VertAng : Outport  Port=74  OutDataTypeStr=single  PortDimensions=1
  Spots8TrackingInfo : Outport  Port=75  OutDataTypeStr=boolean  PortDimensions=1
  Spots8VehObjClassn : Outport  Port=76  OutDataTypeStr=uint8  PortDimensions=1
  SpotsLSVDistance : Outport  Port=77  PortDimensions=6
  SpotsLSV_Types : Outport  Port=78  PortDimensions=6
  wires:
  LSV_valid_state/1 -> Subsystem1/70(LSV_valid_state)
  Subsystem1/64(SpotsLSV_Types) -> SpotsLSV_Types/1
  Subsystem1/63(SpotsLSVDistance) -> SpotsLSVDistance/1
  Subsystem1/50(Spots8VehObjClassn) -> Spots8VehObjClassn/1
  Subsystem1/66(Spots8TrackingInfo) -> Spots8TrackingInfo/1
  Subsystem1/49(Spot8VertAng) -> Spot8VertAng/1
  Subsystem1/48(Spots8HozLeAngSpd) -> Spots8HozLeAngSpd/1
  Subsystem1/12(Spots8Distance) -> Spots8Distance/1
  Subsystem1/15(Spots8HozlPosnLeAng) -> Spots8HozlPosnLeAng/1
  Subsystem1/14(Spots8HozlPosnRiAng) -> Spots8HozlPosnRiAng/1
  Subsystem1/11(Spots8Typ) -> Spots8Typ/1
  Subsystem1/10(Spots8Valid) -> Spots8Valid/1
  Subsystem1/13(Spots7VehObjClassn) -> Spots7VehObjClassn/1
  Subsystem1/65(Spots7TrackingInfo) -> Spots7TrackingInfo/1
  Subsystem1/46(Spot7VertAng) -> Spot7VertAng/1
  Subsystem1/47(Spots7HozLeAngSpd) -> Spots7HozLeAngSpd/1
  Subsystem1/7(Spots7Distance) -> Spots7Distance/1
  Subsystem1/9(Spots7HozlPosnLeAng) -> Spots7HozlPosnLeAng/1
  Subsystem1/8(Spots7HozlPosnRiAng) -> Spots7HozlPosnRiAng/1
  Subsystem1/6(Spots7Typ) -> Spots7Typ/1
  Subsystem1/5(Spots7Valid) -> Spots7Valid/1
  ObjClassn/12(Spots6VehObjClassn) -> Spots6VehObjClassn/1
  ObjClassn/6(Spots6TrackingInfo) -> Spots6TrackingInfo/1  "Spots6TrackingInfo"
  Subsystem1/61(Spot6VertAng) -> Spot6VertAng/1
  Subsystem1/62(Spots6HozLeAngSpd) -> Spots6HozLeAngSpd/1
  Subsystem1/43(Spots6Distance) -> Spots6Distance/1
  Subsystem1/45(Spots6HozlPosnLeAng) -> Spots6HozlPosnLeAng/1
  Subsystem1/44(Spots6HozlPosnRiAng) -> Spots6HozlPosnRiAng/1
  Subsystem1/42(Spots6Typ) -> Spots6Typ/1
  Subsystem1/41(Spots6Valid) -> Spots6Valid/1
  ObjClassn/11(Spots5VehObjClassn) -> Spots5VehObjClassn/1
  ObjClassn/5(Spots5TrackingInfo) -> Spots5TrackingInfo/1  "Spots5TrackingInfo"
  Subsystem1/59(Spot5VertAng) -> Spot5VertAng/1
  Subsystem1/60(Spots5HozLeAngSpd) -> Spots5HozLeAngSpd/1
  Subsystem1/40(Spots5HozlPosnLeAng) -> Spots5HozlPosnLeAng/1
  Subsystem1/38(Spots5Distance) -> Spots5Distance/1
  Subsystem1/39(Spots5HozlPosnRiAng) -> Spots5HozlPosnRiAng/1
  Subsystem1/37(Spots5Typ) -> Spots5Typ/1
  Subsystem1/36(Spots5Valid) -> Spots5Valid/1
  Subsystem1/2(RoadIllumDetd) -> RoadIllumDetd/1
  Subsystem1/1(AmBlight) -> AmBlight/1
  ObjClassn/10(Spots4VehObjClassn) -> Spots4VehObjClassn/1
  ObjClassn/4(Spots4TrackingInfo) -> Spots4TrackingInfo/1  "Spots4TrackingInfo"
  Subsystem1/58(Spots4HozLeAngSpd) -> Spots4HozLeAngSpd/1
  Subsystem1/57(Spot4VertAng) -> Spot4VertAng/1
  Subsystem1/33(Spots4Distance) -> Spots4Distance/1
  Subsystem1/35(Spots4HozlPosnLeAng) -> Spots4HozlPosnLeAng/1
  Subsystem1/34(Spots4HozlPosnRiAng) -> Spots4HozlPosnRiAng/1
  Subsystem1/32(Spots4Typ) -> Spots4Typ/1
  Subsystem1/31(Spots4Valid) -> Spots4Valid/1
  ObjClassn/9(Spots3VehObjClassn) -> Spots3VehObjClassn/1
  ObjClassn/3(Spots3TrackingInfo) -> Spots3TrackingInfo/1  "Spots3TrackingInfo"
  Subsystem1/55(Spot3VertAng) -> Spot3VertAng/1
  Subsystem1/56(Spots3HozLeAngSpd) -> Spots3HozLeAngSpd/1
  Subsystem1/28(Spots3Distance) -> Spots3Distance/1
  Subsystem1/30(Spots3HozlPosnLeAng) -> Spots3HozlPosnLeAng/1
  Subsystem1/29(Spots3HozlPosnRiAng) -> Spots3HozlPosnRiAng/1
  Subsystem1/27(Spots3Typ) -> Spots3Typ/1
  Subsystem1/26(Spots3Valid) -> Spots3Valid/1
  ObjClassn/8(Spots2VehObjClassn) -> Spots2VehObjClassn/1
  ObjClassn/2(Spots2TrackingInfo) -> Spots2TrackingInfo/1  "Spots2TrackingInfo"
  Subsystem1/53(Spot2VertAng) -> Spot2VertAng/1
  Subsystem1/54(Spots2HozLeAngSpd) -> Spots2HozLeAngSpd/1
  Subsystem1/23(Spots2Distance) -> Spots2Distance/1
  Subsystem1/25(Spots2HozlPosnLeAng) -> Spots2HozlPosnLeAng/1
  Subsystem1/24(Spots2HozlPosnRiAng) -> Spots2HozlPosnRiAng/1
  Subsystem1/22(Spots2Typ) -> Spots2Typ/1
  Subsystem1/21(Spots2Valid) -> Spots2Valid/1
  Subsystem1/20(Spots1HozlPosnLeAng) -> Spots1HozlPosnLeAng/1
  Subsystem1/19(Spots1HozlPosnRiAng) -> Spots1HozlPosnRiAng/1
  Subsystem1/18(Spots1Distance) -> Spots1Distance/1
  Subsystem1/17(Spots1Typ) -> Spots1Typ/1
  Subsystem1/16(Spots1Valid) -> Spots1Valid/1
  ObjClassn/7(Spots1VehObjClassn) -> Spots1VehObjClassn/1
  ObjClassn/1(Spots1TrackingInfo) -> Spots1TrackingInfo/1  "Spots1TrackingInfo"
  Subsystem1/51(Spot1VertAng) -> Spot1VertAng/1
  Subsystem1/52(Spots1HozLeAngSpd) -> Spots1HozLeAngSpd/1
  Subsystem1/4(CamerSts) -> CamerSts/1
  Subsystem1/3(TrafficStyle) -> Trafficstyle/1
  LSV_Consecutive_Detection5/1 -> ObjClassn/5(LSV_Consecutive_Detection5)
  LSV_Consecutive_Detection2/1 -> ObjClassn/2(LSV_Consecutive_Detection2)
  LSV_Type2/1 -> Subsystem1/17(LSV_Type2), ObjClassn/20(LSV_Type2)
  LSV_Angular_Velocity_Right6/1 -> Subsystem1/58(LSV_Angular_Velocity_Right6)
  LSV_Left_Angle5/1 -> Subsystem1/47(LSV_Left_Angle5)
  LSV_Right_Angle4/1 -> Subsystem1/37(LSV_Right_Angle4)
  LSV_Sub_Type4/1 -> ObjClassn/13(LSV_Sub_Type4)
  LSV_Top_Angle6/1 -> Subsystem1/57(LSV_Top_Angle6)
  LSV_Angular_Velocity_Left1/1 -> Subsystem1/14(LSV_Angular_Velocity_Left1)
  LSV_CL_Sub_Type4/1 -> ObjClassn/14(LSV_CL_Sub_Type4)
  LSV_Distance6/1 -> Subsystem1/54(LSV_Distance6)
  LSV_Angular_Velocity_Right3/1 -> Subsystem1/31(LSV_Angular_Velocity_Right3)
  LSV_Consecutive_Detection6/1 -> ObjClassn/6(LSV_Consecutive_Detection6)
  LSV_Type6/1 -> Subsystem1/53(LSV_Type6), ObjClassn/24(LSV_Type6)
  LSV_Type1/1 -> Subsystem1/8(LSV_Type1), ObjClassn/19(LSV_Type1)
  LSV_Sub_Type5/1 -> ObjClassn/15(LSV_Sub_Type5)
  LSV_Angular_Velocity_Right5/1 -> Subsystem1/49(LSV_Angular_Velocity_Right5)
  LSV_Consecutive_Detection1/1 -> ObjClassn/1(LSV_Consecutive_Detection1)
  LSR_Distance2/1 -> Subsystem1/66(LSR_Distance2)
  LSV_Top_Angle4/1 -> Subsystem1/39(LSV_Top_Angle4)
  LSV_Angular_Velocity_Right4/1 -> Subsystem1/40(LSV_Angular_Velocity_Right4)
  LSR_Right_Angle2/1 -> Subsystem1/67(LSR_Right_Angle2)
  LSV_Is_New2/1 -> Terminator10/1
  LSR_Top_Angle1/1 -> Subsystem1/64(LSR_Top_Angle1)
  LSV_Angular_Velocity_Left6/1 -> Subsystem1/59(LSV_Angular_Velocity_Left6)
  LSR_ID2/1 -> Subsystem1/65(LSR_ID2)
  LSV_ID6/1 -> Subsystem1/51(LSV_ID6)
  LSV_CL_Sub_Type5/1 -> ObjClassn/16(LSV_CL_Sub_Type5)
  LSV_Right_Angle6/1 -> Subsystem1/55(LSV_Right_Angle6)
  LSR_Left_Angle1/1 -> Subsystem1/63(LSR_Left_Angle1)
  LSV_Left_Angle6/1 -> Subsystem1/56(LSV_Left_Angle6)
  ADB_error/1 -> Subsystem1/2(ADB_error)
  LSV_Distance5/1 -> Subsystem1/45(LSV_Distance5)
  LSV_Distance4/1 -> Subsystem1/36(LSV_Distance4)
  LSV_ID4/1 -> Subsystem1/33(LSV_ID4)
  LSV_Type5/1 -> Subsystem1/44(LSV_Type5), ObjClassn/23(LSV_Type5)
  LSV_Confidence5/1 -> Subsystem1/43(LSV_Confidence5)
  LSV_Type4/1 -> Subsystem1/35(LSV_Type4), ObjClassn/22(LSV_Type4)
  LSV_Angular_Velocity_Left4/1 -> Subsystem1/41(LSV_Angular_Velocity_Left4)
  LSR_Distance1/1 -> Subsystem1/61(LSR_Distance1)
  LSV_Confidence3/1 -> Subsystem1/25(LSV_Confidence3)
  LSV_Type3/1 -> Subsystem1/26(LSV_Type3), ObjClassn/21(LSV_Type3)
  LSV_Distance3/1 -> Subsystem1/27(LSV_Distance3)
  LSV_Confidence2/1 -> Subsystem1/16(LSV_Confidence2)
  LSV_Right_Angle3/1 -> Subsystem1/28(LSV_Right_Angle3)
  LSV_Confidence6/1 -> Subsystem1/52(LSV_Confidence6)
  LSV_ID3/1 -> Subsystem1/24(LSV_ID3)
  LSV_Left_Angle2/1 -> Subsystem1/20(LSV_Left_Angle2)
  LSV_Left_Angle3/1 -> Subsystem1/29(LSV_Left_Angle3)
  LSV_Right_Angle1/1 -> Subsystem1/10(LSV_Right_Angle1)
  LSV_HLB_Reason/1 -> Subsystem1/5(LSV_HLB_Reason)
  LSV_Running_Mode/1 -> Subsystem1/3(LSV_Running_Mode)
  LSV_Top_Angle5/1 -> Subsystem1/48(LSV_Top_Angle5)
  LSV_Confidence1/1 -> Subsystem1/7(LSV_Confidence1)
  LSV_Angular_Velocity_Left3/1 -> Subsystem1/32(LSV_Angular_Velocity_Left3)
  VehConfigADB/1 -> Subsystem1/1(VehConfigADB)
  LSV_CL_Sub_Type6/1 -> ObjClassn/18(LSV_CL_Sub_Type6)
  LSV_Sub_Type2/1 -> ObjClassn/9(LSV_Sub_Type2)
  LSV_Confidence4/1 -> Subsystem1/34(LSV_Confidence4)
  LSV_Consecutive_Detection4/1 -> ObjClassn/4(LSV_Consecutive_Detection4)
  LSV_Sub_Type1/1 -> ObjClassn/7(LSV_Sub_Type1)
  LSV_Distance1/1 -> Subsystem1/9(LSV_Distance1)
  LSV_Distance2/1 -> Subsystem1/18(LSV_Distance2)
  LSV_Is_New6/1 -> Terminator38/1
  LSV_Is_New1/1 -> Terminator3/1
  LSV_Sub_Type6/1 -> ObjClassn/17(LSV_Sub_Type6)
  LSV_Right_Angle2/1 -> Subsystem1/19(LSV_Right_Angle2)
  LSV_Top_Angle2/1 -> Subsystem1/21(LSV_Top_Angle2)
  LSV_Left_Angle1/1 -> Subsystem1/11(LSV_Left_Angle1)
  LSV_Is_New3/1 -> Terminator17/1
  LSV_ID2/1 -> Subsystem1/15(LSV_ID2)
  LSV_Angular_Velocity_Right2/1 -> Subsystem1/22(LSV_Angular_Velocity_Right2)
  LSR_Left_Angle2/1 -> Subsystem1/68(LSR_Left_Angle2)
  LSV_ID1/1 -> Subsystem1/6(LSV_ID1)
  LSR_Right_Angle1/1 -> Subsystem1/62(LSR_Right_Angle1)
  LSV_ID5/1 -> Subsystem1/42(LSV_ID5)
  LSV_CL_Sub_Type1/1 -> ObjClassn/8(LSV_CL_Sub_Type1)
  LSV_Angular_Velocity_Left5/1 -> Subsystem1/50(LSV_Angular_Velocity_Left5)
  LSV_Is_New5/1 -> Terminator31/1
  LSV_Consecutive_Detection3/1 -> ObjClassn/3(LSV_Consecutive_Detection3)
  LSV_Right_Angle5/1 -> Subsystem1/46(LSV_Right_Angle5)
  LSV_Top_Angle1/1 -> Subsystem1/12(LSV_Top_Angle1)
  LSV_CL_Sub_Type3/1 -> ObjClassn/12(LSV_CL_Sub_Type3)
  LSV_Sub_Type3/1 -> ObjClassn/11(LSV_Sub_Type3)
  LSV_Top_Angle3/1 -> Subsystem1/30(LSV_Top_Angle3)
  LSR_Top_Angle2/1 -> Subsystem1/69(LSR_Top_Angle2)
  LSV_Angular_Velocity_Right1/1 -> Subsystem1/13(LSV_Angular_Velocity_Right1)
  LSV_HLB_Decision/1 -> Subsystem1/4(LSV_HLB_Decision)
  LSV_Is_New4/1 -> Terminator24/1
  LSV_Angular_Velocity_Left2/1 -> Subsystem1/23(LSV_Angular_Velocity_Left2)
  LSV_CL_Sub_Type2/1 -> ObjClassn/10(LSV_CL_Sub_Type2)
  LSR_ID1/1 -> Subsystem1/60(LSR_ID1)
  LSV_Left_Angle4/1 -> Subsystem1/38(LSV_Left_Angle4)
